simulink model "CubeX_LQR_2D"  (R2016b)
settings: Solver=FixedStepDiscrete  StartTime=0.0  StopTime=inf  FixedStep=Ts.base  RelTol=1e-3
PreLoadFcn:
  | waijung.modelPreload; % Required for working with Waijung Blockset. Do not remove.
InitFcn:
  | cubeparameters
  | LQR_2d
undefined symbols (not defined in the file): CPHA_1Edge, CPOL_Low, deg_, Duplex, FirstBit_MSB, Full, g, imu, K_lqr, Link, LQFP100, ST, STM32F407VG, STM32F4DISCOVERY, Ts
libraries: simulink x58, stm32f4_i2c_lib x12, stm32f4_io_lib x6, cube_lib x4, stm32f4_spi_lib x4, stm32f4_adc_lib x1, stm32f4_device_config_lib x1, BC_USB x1
(part 1 of 4)
CloseFcn:
  | waijung.modelClose; % Required for working with Waijung Blockset. Do not remove.
settings Model: Creator=Hi  LastModifiedBy=Wall
settings DataIOCC: LimitDataPoints=on  SaveFormat=Array
settings OptimizationCC: LifeSpan=1
settings DebuggingCC: AllowSymbolicDim=off  SFUnexpectedBacktrackingDiag=warning  SFNoUnconditionalDefaultTransitionDiag=warning  SFExecutionAtInitializationDiag=none
settings HardwareCC: ProdBitPerPointer=32  ProdBitPerSizeT=32  ProdBitPerPtrDiffT=32  ProdLargestAtomicFloat=None  ProdIntDivRoundTo=Undefined  ProdWordSize=32  ProdHWDeviceType=ARM Compatible->Cortex - M4  TargetEndianess=LittleEndian  TargetHWDeviceType=ARM Compatible->Cortex - M4
settings ModelReferenceCC: PropagateSignalLabelsOutOfModel=off
settings RTWCC: SystemTargetFile=stm32f4.tlc  GenerateMakefile=off  TemplateMakefile=ert_default_tmf  Description=STM32F4 Target
settings CodeAppCC: ForceParamTrailComments=on  IgnoreCustomStorageClasses=off  OperatorAnnotations=on  SimulinkDataObjDesc=on  InsertBlockDesc=on  MATLABSourceComments=on
settings STFCustomTargetCC: ModelReferenceCompliant=off  CombineOutputUpdateFcns=on  ERTCustomFileBanners=on  SupportContinuousTime=off  SupportNonInlinedSFcns=off  RemoveResetFunc=on  MATLABClassNameForMDSCustomization=Simulink.SoftwareTarget.ERTCustomization  GRTInterface=off  SystemTargetFile=stm32f4.tlc
settings ERTTargetCC: ModelReferenceCompliant=off  ParMdlRefBuildCompliant=off  CompOptLevelCompliant=off  ConcurrentExecutionCompliant=off  ERTFirstTimeCompliant=off  ModelStepFunctionPrototypeControlCompliant=off  CPPClassGenCompliant=off  UseToolchainInfoCompliant=off  ERTSrcFileBannerTemplate=stm32f4_code_template.cgt  ERTHdrFileBannerTemplate=stm32f4_code_template.cgt  ERTDataSrcFileTemplate=stm32f4_code_template.cgt  ERTDataHdrFileTemplate=stm32f4_code_template.cgt  ERTCustomFileTemplate=stm32f4_file_process.tlc  ConvertIfToSwitch=off  SuppressUnreachableDefaultCases=off
settings ConfigComp: CovMetricSettings=dw  CovHtmlReporting=on  CovSaveCumulativeToWorkspaceVar=on  CovSaveSingleToWorkspaceVar=on  CovExternalEMLEnable=off

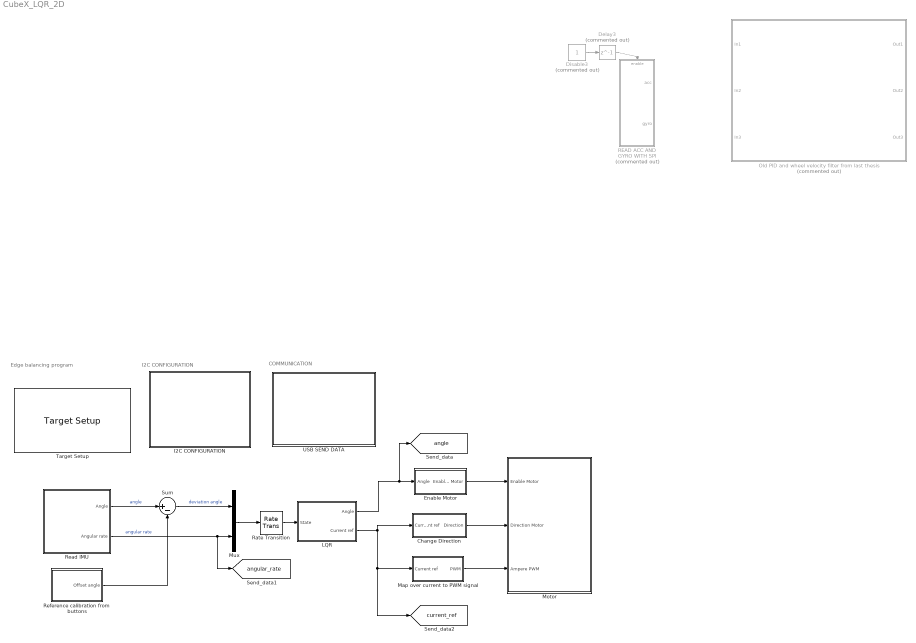
== system CubeX_LQR_2D ==
  note: Edge balancing program
  note: COMMUNICATION
  note: I2C CONFIGURATION
  Change Direction : Subsystem
  Delay3 : Delay  Commented=on  DelayLength=1  InitialCondition=0
  Disable3 : Constant  Commented=on
  Enable Motor : Subsystem  SystemSampleTime=Ts.controller
  I2C CONFIGURATION : Subsystem
  LQR : Subsystem  SystemSampleTime=Ts.controller
      settings: MinAlgLoopOccurrences=on
  Map over current to PWM signal : Subsystem
  Motor : Subsystem
  Mux : Mux  Inputs=2
  Old PID and wheel velocity filter from last thesis : Subsystem  Commented=on
  READ ACC AND GYRO WITH SPI : Subsystem  Commented=on
  Rate Transition : RateTransition  OutPortSampleTime=Ts.controller
  Read IMU : Subsystem
  Reference calibration from buttons : Subsystem
  Sum : Sum  Inputs=|+-
  Target Setup : stm32f4_device_config_lib/Target Setup  Priority=100  compiler=GNU ARM  previous_compiler=GNU ARM  mcu=STM32F407VG (LQFP100); STM32F4DISCOVERY  mcustr=STM32F407VG  clockconfig=STM32F4DISCOVERY Default (HSEOSC-8MHz/HCLK-168MHz)  system_stm32f4xx_c_path=C:\waijung15_04a\targets\stm32f4_target\stm32f4\utils\STM32F4xx_AN3988_V1.0.1\stm32f4_default\hseosc8mhz  showmemoryconfiguration=off  stacksize=0x400  heapsize=0x200  enableautocompiledownload=on  fullchiperase=off  programmerinterface=ST-Link  editctrlstr=on  compilercontrolstr=$(patsubst %, -I%, .) -mcpu=cortex-m4 -mthumb -mthumb-interwork -mfloat-abi=hard -mfpu=fpv4-sp-d16 -ffast-math -Wall -Wextra -Ofast  assemblercontrolstr=$(patsubst %, -I%, .) -mcpu=cortex-m4 -mthumb -mthumb-interwork -mfloat-abi=hard -mfpu=fpv4-sp-d16 -ffast-math -Wall -Wextra -Ofast -Wa,-amhls=$(<:.s=.lst) -D__STACK_SIZE=$(STACK_SIZE) -D__HEAP_SIZE=$(HEAP_SIZE)  linkercontrolstr=-T$(LD_SCRIPT) -g -Wl,-Map=$(MAP),--cref,--no-warn-mismatch -mcpu=cortex-m4 -mthumb -mthumb-interwork -mfloat-abi=hard -mfpu=fpv4-sp-d16  runafterdownload=on  execprofile=None  profileruart=1  profilerbaud=115200  profilertxpin=Not used  profilerinitstr=0.002,168000000,336000,115200,0  manualsetsampletime=on  sampletime=0.002  blockid=TargetSetup1  systickreloadvalue=336000  hseval=8000000  lastprofileruart=1  hclk=168000000  flashorigin=0x8000000  flashlength=1M  ramorigin=0x20000000  ramlength=112k  useextram=off
  USB SEND DATA : Subsystem
  tag scope: angle=global, angular_rate=global, current_ref=global
  wires:
  Disable3/1 -> Delay3/1
  Delay3/1 -> READ ACC AND GYRO WITH SPI/Enable
  Read IMU/2(Angular rate) -> [angular_rate], Mux/2  "angular rate"
  Reference calibration from buttons/1(Offset angle) -> Sum/2
  Sum/1 -> Mux/1  "deviation angle"
  Read IMU/1(Angle) -> Sum/1  "angle"
  LQR/2(Current ref) -> [current_ref], Map over current to PWM signal/1(Current ref), Change Direction/1(Current ref)
  Map over current to PWM signal/1(PWM) -> Motor/3(Ampere PWM)
  Change Direction/1(Direction) -> Motor/2("Direction Motor ")
  Enable Motor/1(Enable Motor) -> Motor/1(Enable Motor)
  Mux/1 -> Rate Transition/1
  Rate Transition/1 -> LQR/1(State)
  LQR/1(Angle) -> [angle], Enable Motor/1(Angle)

== system CubeX_LQR_2D/Change Direction ==
  Current ref : Inport
  Compare To Zero : simulink/Logic and Bit Operations/Compare To Zero  relop=<=  OutDataTypeStr=boolean
  Logical Operator : Logic  Operator=NOT  AllPortsSameDT=off  OutDataTypeStr=boolean
  Direction : Outport
  wires:
  Compare To Zero/1 -> Logical Operator/1
  Current ref/1 -> Compare To Zero/1
  Logical Operator/1 -> Direction/1

== system CubeX_LQR_2D/Enable Motor ==
  note: When the angle is abs of 6 degrees, Motor is enabled
  Angle : Inport
  Abs1 : Abs
  Compare To Constant : simulink/Logic and Bit Operations/Compare To Constant  relop=<=  const=deg2rad(3)  OutDataTypeStr=boolean
  Enable Motor : Outport
  wires:
  Abs1/1 -> Compare To Constant/1
  Angle/1 -> Abs1/1
  Compare To Constant/1 -> Enable Motor/1

== system CubeX_LQR_2D/I2C CONFIGURATION ==
  I2C Master Setup1 : S-Function  FunctionName=stm32f4_i2c  Parameters=configuration,module,transfer,clkspeed,timeout,sdapin,sclpin,writecount,readcount,inputtypearray,outputtypearray,confstr,sampletime,sampletimestr,blockid  SFunctionDeploymentMode=off  EnableBusSupport=off  mask(stm32f4_i2c){configuration=Setup, module=3, lastmodule=3, transfer=Blocking, dutycycle=TLow/THigh = 2, clkspeed=400, timeout=25, writecount=0, readcount=0, sdapin=C9, sclpin=A8, waitwritetime=0, inputtypearray=[0], outputtypearray=[0], confstr=["C","9","A","8","1","3","4","2","I2C_DutyCycle_2","0","off"], sampletime=-1, sampletimestr=0.002, blockid=I2CCONFIGURATIONI2CMasterSetup1}
      mask prompts: module "I2C Module"; lastmodule "Last module"; transfer "Transfer mode"; dutycycle "Duty cycle in fast mode"; clkspeed "Clock speed (kHz)"; timeout "Timeout (ms)"; writecount "Bytes write count"; readcount "Bytes read count"; sdapin "SDA pin"; sclpin "SCL pin"; waitwritetime "Wait write time (ms), default is 0"; inputtypearray "Input type array"; outputtypearray "Output type array"; confstr "Configuration string"; sampletime "Sample time (sec)"; sampletimestr "Compiled sample time (sec) in string"
      mask init:
      | stm32f4_i2c_callback('init');
      mask Help: web(fullfile(waijungdocroot,'stm32f4_i2c_setup.htm'), '-browser')
      mask TypeOptions configuration: Setup | Transaction
      mask Callback configuration: stm32f4_i2c_callback('configuration');
      mask TypeOptions module: 1 | 2 | 3
      mask Callback module: stm32f4_i2c_callback('module');
      mask TypeOptions transfer: Blocking | Non-blocking
      mask TypeOptions dutycycle: TLow/THigh = 16/9 | TLow/THigh = 2
      mask Callback dutycycle: stm32f4_i2c_callback('dutycycle');
      mask Callback writecount: stm32f4_i2c_callback('writecount');
      mask Callback readcount: stm32f4_i2c_callback('readcount');
      mask TypeOptions sdapin: - | C9
      mask Callback sdapin: stm32f4_i2c_callback('sdapin');
      mask TypeOptions sclpin: - | A8
      mask Callback sclpin: stm32f4_i2c_callback('sclpin');
      mask Callback confstr: stm32f4_i2c_callback('confstr');
      mask Callback sampletime: stm32f4_i2c_callback('sampletime');
      mask Callback sampletimestr: stm32f4_i2c_callback('sampletimestr');
      mask Callback blockid: stm32f4_i2c_callback('blockid');
      mask Display: text(0.5, 0.5, 'Module: I2C3\nClock: 400kHz\nSDA/SCL Pin: C9/A8','ver','middle','hor','center');
  I2C Master Setup2 : S-Function  FunctionName=stm32f4_i2c  Parameters=configuration,module,transfer,clkspeed,timeout,sdapin,sclpin,writecount,readcount,inputtypearray,outputtypearray,confstr,sampletime,sampletimestr,blockid  SFunctionDeploymentMode=off  EnableBusSupport=off  mask(stm32f4_i2c){configuration=Setup, module=1, lastmodule=1, transfer=Blocking, dutycycle=TLow/THigh = 2, clkspeed=400, timeout=25, writecount=0, readcount=0, sdapin=B9, sclpin=B6, waitwritetime=0, inputtypearray=[0], outputtypearray=[0], confstr=["B","9","B","6","1","1","6","0","I2C_DutyCycle_2","0","off"], sampletime=-1, sampletimestr=0.002, blockid=I2CCONFIGURATIONI2CMasterSetup2}
      mask prompts: module "I2C Module"; lastmodule "Last module"; transfer "Transfer mode"; dutycycle "Duty cycle in fast mode"; clkspeed "Clock speed (kHz)"; timeout "Timeout (ms)"; writecount "Bytes write count"; readcount "Bytes read count"; sdapin "SDA pin"; sclpin "SCL pin"; waitwritetime "Wait write time (ms), default is 0"; inputtypearray "Input type array"; outputtypearray "Output type array"; confstr "Configuration string"; sampletime "Sample time (sec)"; sampletimestr "Compiled sample time (sec) in string"
      mask init:
      | stm32f4_i2c_callback('init');
      mask Help: web(fullfile(waijungdocroot,'stm32f4_i2c_setup.htm'), '-browser')
      mask TypeOptions configuration: Setup | Transaction
      mask Callback configuration: stm32f4_i2c_callback('configuration');
      mask TypeOptions module: 1 | 2 | 3
      mask Callback module: stm32f4_i2c_callback('module');
      mask TypeOptions transfer: Blocking | Non-blocking
      mask TypeOptions dutycycle: TLow/THigh = 16/9 | TLow/THigh = 2
      mask Callback dutycycle: stm32f4_i2c_callback('dutycycle');
      mask Callback writecount: stm32f4_i2c_callback('writecount');
      mask Callback readcount: stm32f4_i2c_callback('readcount');
      mask TypeOptions sdapin: - | B7 | B9
      mask Callback sdapin: stm32f4_i2c_callback('sdapin');
      mask TypeOptions sclpin: - | B6 | B8
      mask Callback sclpin: stm32f4_i2c_callback('sclpin');
      mask Callback confstr: stm32f4_i2c_callback('confstr');
      mask Callback sampletime: stm32f4_i2c_callback('sampletime');
      mask Callback sampletimestr: stm32f4_i2c_callback('sampletimestr');
      mask Callback blockid: stm32f4_i2c_callback('blockid');
      mask Display: text(0.5, 0.5, 'Module: I2C1\nClock: 400kHz\nSDA/SCL Pin: B9/B6','ver','middle','hor','center');

== system CubeX_LQR_2D/LQR ==
  note: State feedback
      |
      | u = -Kx
  State : Inport
  Delay : Delay  DelayLength=1
  Demux : Demux  Outputs=2
  Estimate COG offset : MATLAB Function  TreatAsAtomicUnit=on
  Gain : Gain  Gain=-K_lqr  Multiplication=Matrix(K*u) (u vector)
  Mux : Mux  Inputs=2
  Sum : Sum  Inputs=++|
  Angle : Outport
  Current ref : Outport  Port=2
  tag scope: cog=global
  wires:
  Gain/1 -> Current ref/1, Estimate COG offset/1(iref)
  Demux/2 -> Mux/2, Estimate COG offset/3(wx)
  State/1 -> Demux/1
  Mux/1 -> Gain/1
  Sum/1 -> Angle/1, Mux/1
  Estimate COG offset/1(y) -> Delay/1
  Demux/1 -> Sum/2, Estimate COG offset/2(phi)
  Delay/1 -> Sum/1, [cog]

== system CubeX_LQR_2D/Map over current to PWM signal ==
  note: Debug for static friction
  note: Map over current to duty
      | current limit: 0-4A
      | duty limit: 10-90%
      |
      | (90-10) / (4-0) = 20 -> k
      | 10 -> m
  Current ref : Inport
  Abs : Abs
  Add : Sum
  Constant : Constant  Value=0  OutDataTypeStr=single  SampleTime=Ts.controller
  Saturation on duty : Saturate  UpperLimit=90  LowerLimit=10  OutDataTypeStr=single
  Sum : Sum  Inputs=|++
  k : Gain  Gain=20
  m : Constant  Value=10  OutDataTypeStr=single  SampleTime=Ts.controller
  PWM : Outport
  wires:
  Saturation on duty/1 -> PWM/1
  Current ref/1 -> Abs/1
  Abs/1 -> k/1
  k/1 -> Add/1
  m/1 -> Add/2
  Add/1 -> Sum/1
  Sum/1 -> Saturation on duty/1
  Constant/1 -> Sum/2

== system CubeX_LQR_2D/Motor ==
  Enable Motor : Inport
  "Direction Motor " : Inport  Port=2
  Ampere PWM : Inport  Port=3
  Direction Motor 3 (green) : stm32f4_io_lib/Digital Output  use_bitband=on  port=D  speed=100  porttype=Push Pull  porttypestr=PP  use_pin0=off  use_pin1=off  use_pin2=off  use_pin3=off  use_pin4=off  use_pin5=off  use_pin6=off  use_pin7=off  use_pin8=off  use_pin9=off  use_pin10=off  use_pin11=on  use_pin12=off  use_pin13=off  use_pin14=off  use_pin15=off  pinstr=GPIO_Pin_11  usedpinarray="[0  0  0  0  0  0  0  0  0  0  0  1  0  0  0  0]"  bitbandingstr="#define Motor1DirectionMotor3green_D11 Peripheral_BB(GPIOD->ODR, 11)  /* Output pin */"  sampletime=-1  sampletimestr=0.016  blockid=Motor1DirectionMotor3green  enablecustomportlabel=off  globalinit=off  cinputportlabel=In1, In2  coutputportlabel=0
  Enable Motor 3(yellow) : stm32f4_io_lib/Digital Output  use_bitband=on  port=D  speed=100  porttype=Push Pull  porttypestr=PP  use_pin0=off  use_pin1=off  use_pin2=off  use_pin3=off  use_pin4=off  use_pin5=off  use_pin6=off  use_pin7=off  use_pin8=off  use_pin9=on  use_pin10=off  use_pin11=off  use_pin12=off  use_pin13=off  use_pin14=off  use_pin15=off  pinstr=GPIO_Pin_9  usedpinarray="[0  0  0  0  0  0  0  0  0  1  0  0  0  0  0  0]"  bitbandingstr="#define Motor1EnableMotor3yellow_D9 Peripheral_BB(GPIOD->ODR, 9)  /* Output pin */"  sampletime=-1  sampletimestr=0.016  blockid=Motor1EnableMotor3yellow  enablecustomportlabel=off  globalinit=off  cinputportlabel=In1, In2  coutputportlabel=0
  PWM Ampere motor 3 : S-Function  FunctionName=stm32f4_basicpwm_fixed  Parameters=timer,pwmperiod,uc3m_pwmperiod,ch1pin,ch2pin,ch3pin,ch4pin,sampletime,sampletimestr,blockid,apb,portstr,pinstr,pinmat,timarr,timprescale,chmat,polaritystr  SFunctionDeploymentMode=off  EnableBusSupport=off  mask(stm32f4_basicpwm_fixed){timer=2, pwmperiod=0.02, uc3m_pwmperiod=0.0002, polarity=Active High, polaritystr=TIM_OCPolarity_High, ch1pin=Not available - Do not use, ch2pin=Not available - Do not use, ch3pin=Not available - Do not use, ch4pin=A3, sampletime=-1, sampletimestr=0.016, blockid=Motor1PWMAmperemotor3, portpinstr=,,,A3, enablecustomportlabel=off, cinputportlabel=In1, In2, In3, In4, coutputportlabel=0, callbackgensrccode=off, apb=1, portstr=["A"], pinstr=["GPIO_Pin_3"], pinmat=[1 3], timarr=59999, timprescale=55, chmat=[4]}
      mask prompts: pwmperiod "PWM Period (seconds)"; uc3m_pwmperiod "PWM Signal Period (seconds)"; ch1pin "Channel 1"; ch2pin "Channel 2"; ch3pin "Channel 3"; ch4pin "Channel 4"; sampletime "Sample time (sec)"; sampletimestr "Compiled sample time (sec) in string"; portpinstr "Port pin string"; enablecustomportlabel "Enable custom port labels"; cinputportlabel "Custom input port labels (Ex. In1, In2, In3)"; coutputportlabel "Custom output port labels (Ex. Out1, Out2, Out3)"; callbackgensrccode "Gen source code from callback"; portstr "Port string"; pinstr "Pin string"; pinmat "Pin matrix"; timarr "Timer ARR"; timprescale "Timer PRESCALE"; chmat "Channel order"
      mask help:
      | This block implements basic Edge-aligned Pulse Width Modulation (PWM) generation.
      | All timers are 16-bit. The PWM period is fixed (per timer).
      |
      | This block was fixed by Sr Antonio
      mask init:
      | stm32f4_basicpwm_callback_fixed('init');
      mask Help: web(fullfile(waijungdocroot,'stm32f4_basicpwm.htm'),'-browser')
      mask TypeOptions timer: 1 | 2 | 3 | 4 | 5 | 8 | 9 | 10 | 11 | 12 | 13 | 14
      mask Callback timer: stm32f4_basicpwm_callback_fixed('timer');
      mask Callback pwmperiod: stm32f4_basicpwm_callback_fixed('pwmperiod');
      mask Callback uc3m_pwmperiod: stm32f4_basicpwm_callback_fixed('uc3m_pwmperiod');
      mask TypeOptions polarity: Active High | Active Low
      mask Callback polarity: stm32f4_basicpwm_callback_fixed('polarity');
      mask TypeOptions ch1pin: Not available - Do not use | A0 | A5
      mask Callback ch1pin: stm32f4_basicpwm_callback_fixed('ch1pin');
      mask TypeOptions ch2pin: Not available - Do not use | A1 | B3
      mask Callback ch2pin: stm32f4_basicpwm_callback_fixed('ch2pin');
      mask TypeOptions ch3pin: Not available - Do not use | A2 | B10
      mask Callback ch3pin: stm32f4_basicpwm_callback_fixed('ch3pin');
      mask TypeOptions ch4pin: Not available - Do not use | A3 | B11
      mask Callback ch4pin: stm32f4_basicpwm_callback_fixed('ch4pin');
      mask Callback sampletime: stm32f4_basicpwm_callback_fixed('sampletime');
      mask Callback sampletimestr: stm32f4_basicpwm_callback_fixed('sampletimestr');
      mask Callback blockid: stm32f4_basicpwm_callback_fixed('blockid');
      mask Callback enablecustomportlabel: stm32f4_basicpwm_callback_fixed('enablecustomportlabel')
      mask Display: text(0.95, 0.5, 'UC3M FIXED\nTimer: 2\nPolarity: Active High\nPeriod (sec): 0.0002\nTs (sec): -1','ver','middle','hor','right');port_label('input', 1,'CH4 (A3)')
  "Velocty wheel 3, analog in (Grey), PC1" : stm32f4_adc_lib/Regular ADC  Commented=on  adcmodule=3  outputdatatype=Single  prescaler=2  prescalerstr=ADC_Prescaler_Div2  chsamplingtime=Auto  chsamplingtimestr=ADC_SampleTime_480Cycles  read_an0=off  read_an1=off  read_an2=off  read_an3=off  read_an4=off  read_an5=off  read_an6=off  read_an7=off  read_an8=off  read_an9=off  read_an10=on  read_an11=off  read_an12=off  read_an13=off  read_an14=off  read_an15=off  read_an16=off  read_an17=off  read_an18=off  pinstr=GPIO_Pin_10  usedpinarray="[0  0  0  0  0  0  0  0  0  0  1  0  0  0  0  0  0  0  0]"  usedportidarray=[2]  usedpinidarray=[0]  usedpinidcount=1  sampletime=0.002  blockid=Motor3Veloctywheel3analoginGreyPC1  enablecustomportlabel=off  cinputportlabel=0  coutputportlabel=Out1, Out2
  wires:
  Ampere PWM/1 -> PWM Ampere motor 3/1
  "Direction Motor "/1 -> Direction Motor 3 (green)/1
  Enable Motor/1 -> Enable Motor 3(yellow)/1

== system CubeX_LQR_2D/Old PID and wheel velocity filter from last thesis ==
  In1 : Inport
  In2 : Inport  Port=2
  In3 : Inport  Port=3
  Filetered Wheel 3 : Subsystem  Commented=on
  "PID Motor 3 DONE " : Subsystem  Commented=on
  Out1 : Outport
  Out2 : Outport  Port=2
  Out3 : Outport  Port=3
  wires:
  In1/1 -> "PID Motor 3 DONE "/1("Welocity Wheel ")
  "PID Motor 3 DONE "/2("Direction_Motor_3 ") -> Out3/1
  In2/1 -> Filetered Wheel 3/1(In1)
  Filetered Wheel 3/1(Out1) -> Out2/1
  "PID Motor 3 DONE "/1(Motor_3_Out) -> Out1/1
  In3/1 -> "PID Motor 3 DONE "/2(Angle)

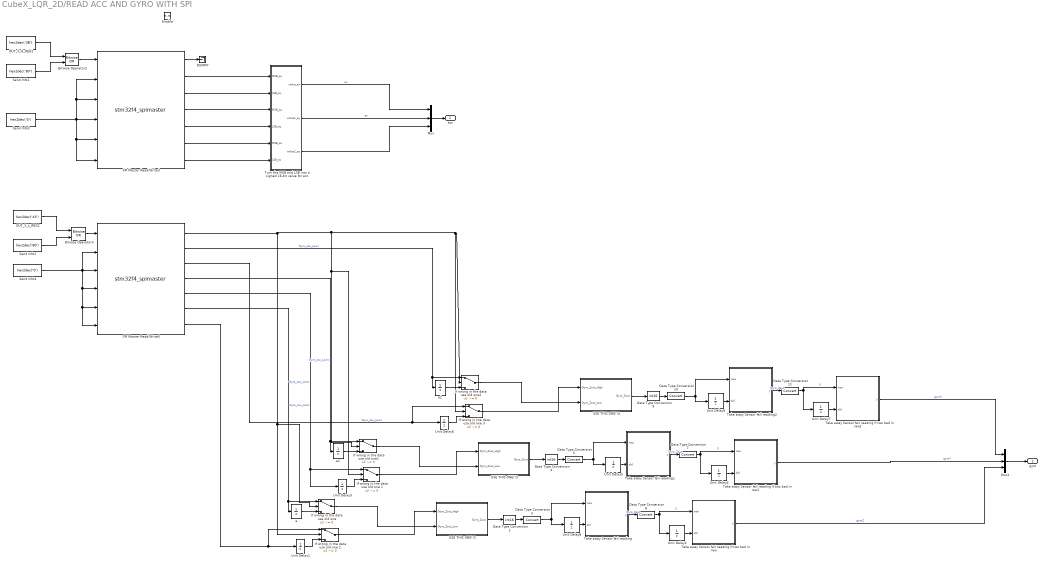
== system CubeX_LQR_2D/READ ACC AND GYRO WITH SPI ==
  Enable : EnablePort
  " a" : UnitDelay  SampleTime=-1
  " a1" : UnitDelay  SampleTime=-1
  " a2" : UnitDelay  SampleTime=-1
  Bitwise Operator2 : simulink/Logic and Bit Operations/Bitwise Operator  logicop=OR  UseBitMask=off  NumInputPorts=2  BitMask=bin2dec('11011001')  BitMaskRealWorld=Stored Integer
  Bitwise Operator3 : simulink/Logic and Bit Operations/Bitwise Operator  logicop=OR  UseBitMask=off  NumInputPorts=2  BitMask=bin2dec('11011001')  BitMaskRealWorld=Stored Integer
  DUMMY : Terminator
  Data Type Conversion{3,5,7..8,10..11} (6 alike) : DataTypeConversion
  Data Type Conversion2 : DataTypeConversion  OutDataTypeStr=int16
  Data Type Conversion4 : DataTypeConversion  OutDataTypeStr=int16
  Data Type Conversion9 : DataTypeConversion  OutDataTypeStr=int16
  If wrong in the data use old one : Switch  Criteria=u2 ~= 0
  If wrong in the data use old one 1 : Switch  Criteria=u2 ~= 0
  If wrong in the data use old one 2 : Switch  Criteria=u2 ~= 0
  If wrong in the data use old one 3 : Switch  Criteria=u2 ~= 0
  If wrong in the data use old one1 : Switch  Criteria=u2 ~= 0
  If wrong in the data use old one2 : Switch  Criteria=u2 ~= 0
  Mux : Mux  Inputs=3
  Mux1 : Mux  Inputs=3
  OUT_X_H_REG1 : Constant  Value=hex2dec('3B')  OutDataTypeStr=uint8
  OUT_X_L_REG2 : Constant  Value=hex2dec('43')  OutDataTypeStr=uint8
  SPI Master Read/Write3 : S-Function  FunctionName=stm32f4_spimaster  Parameters=mode,configuration,module,datacount,inputtypearray,outputtypearray,confstr,sampletime,sampletimestr,blockid  SFunctionDeploymentMode=off  EnableBusSupport=off  mask(stm32f4_spimaster){configuration=Transaction, module=3, mode=Read/ Write, lastmodule=1, direction=Full-Duplex, dataformat=8bit/ FirstBit_MSB, prescaler=4, cpolcpha=CPOL_Low/ CPHA_1Edge, datacount=6, nssmode=Custom, nsspin=Not used, softnssport=E, softnsspin=0, sckpin=A5, misopin=A6, mosipin=A7, inputtypearray=[6 3 3 3 3 3 3], outputtypearray=[7 7 3 3 3 3 3 3], confstr=["SPI_Direction_2Lines_FullDuplex","8b","MSB","Low","1Edge","4","Soft","0","x","x","0","x","x","1","A","5","1","A","6","1","A","7","1","0","0","0","0","0","0","0","0","PP","0","UP"], sampletime=-1, sampletimestr=Inf, blockid=SPI3getData4SPIMasterReadWrite3}
      mask prompts: module "SPI Module:"; lastmodule "Last module:"; dataformat "Data format:"; prescaler "Buad rate prescaler: Pclk/"; cpolcpha "Clock polarity (CPOL)/ Clock phase (CPHA):"; datacount "Data Read/Write count:"; nssmode "Slave/chip select (nSS, nCS) mode"; nsspin "Slave/chip select (nSS, nCS) pin"; softnssport "Slave/chip select port (nSS, nCS)"; softnsspin "Slave/chip select pin (nSS, nCS)"; sckpin "SCLK pin:"; misopin "MISO pin:"; mosipin "MOSI pin:"; inputtypearray "Input type array"; outputtypearray "Output type array"; confstr "Configuration string"; sampletime "Sample time (sec)"; sampletimestr "Compiled sample time (sec) in string"
      mask help:
      | Status:
      |  0 - Success.
      |  Otherwise - Fail.
      mask init:
      | stm32f4_spimaster_callback('init');
      mask Help: web(fullfile(waijungdocroot,'stm32f4_spimaster_readwrite.htm'), '-browser')
      mask TypeOptions configuration: Setup | Transaction
      mask Callback configuration: stm32f4_spimaster_callback('configuration');
      mask TypeOptions module: 1 | 2 | 3
      mask Callback module: stm32f4_spimaster_callback('module');
      mask TypeOptions mode: Read/ Write | Read | Write
      mask Callback mode: stm32f4_spimaster_callback('mode');
      mask TypeOptions direction: Full-Duplex | Half-Duplex_Tx | Half-Duplex_Rx
      mask Callback direction: stm32f4_spimaster_callback('direction');
      mask TypeOptions dataformat: 8bit/ FirstBit_MSB | 8bit/ FirstBit_LSB | 16bit/ FirstBit_MSB | 16bit/ FirstBit_LSB
      mask TypeOptions prescaler: 2 | 4 | 8 | 16 | 32 | 64 | 128 | 256
      mask TypeOptions cpolcpha: CPOL_Low/ CPHA_1Edge | CPOL_Low/ CPHA_2Edge | CPOL_High/ CPHA_1Edge | CPOL_High/ CPHA_2Edge
      mask Callback datacount: stm32f4_spimaster_callback('datacount');
      mask TypeOptions nssmode: Hardware | Software | Custom
      mask Callback nssmode: stm32f4_spimaster_callback('nssmode');
      mask TypeOptions nsspin: Not used | A4 | A15
      mask TypeOptions softnssport: A | B | C | D | E | F | G | H | I
      mask TypeOptions softnsspin: 0 | 1 | 2 | 3 | 4 | 5 | 6 | 7 | 8 | 9 | 10 | 11 | 12 | 13 | 14 | 15
      mask TypeOptions sckpin: Not used | A5 | B3
      mask TypeOptions misopin: Not used | A6 | B4
      mask TypeOptions mosipin: Not used | A7 | B5
      mask Callback confstr: stm32f4_spimaster_callback('confstr');
      mask Callback sampletime: stm32f4_spimaster_callback('sampletime');
      mask Callback sampletimestr: stm32f4_spimaster_callback('sampletimestr');
      mask Callback blockid: stm32f4_spimaster_callback('blockid');
      mask Display: text(0.5, 0.5, 'Module: SPI3 (Master)\nRead/ Write\nTs (sec): Inf','ver','middle','hor','center');port_label('input', 1,'Wr0 (uint8)');port_label('input', 2,'Wr1 (uint8)');port_label('input', 3,'Wr2 (uint8)');port_label('input', 4,'Wr3 (uint8)');port_label('input', 5,'Wr4 (uint8)');port_label('input', 6,'Wr5 (uint8)');port_label('output', 1,'Status');port_label('output', 2,'Rd0 (uint8)');port_label('output', 3,'Rd1 (uint8)');port_label('output', 4,'Rd2 (uint8)');port_label('output', 5,'Rd3 (uint8)');port_label('output', 6,'Rd4 (uint8)');port_label('output', 7,'Rd5 (uint8)');
  SPI Master Read/Write5 : S-Function  FunctionName=stm32f4_spimaster  Parameters=mode,configuration,module,datacount,inputtypearray,outputtypearray,confstr,sampletime,sampletimestr,blockid  SFunctionDeploymentMode=off  EnableBusSupport=off  mask(stm32f4_spimaster){configuration=Transaction, module=3, mode=Read/ Write, lastmodule=1, direction=Full-Duplex, dataformat=8bit/ FirstBit_MSB, prescaler=4, cpolcpha=CPOL_Low/ CPHA_1Edge, datacount=6, nssmode=Custom, nsspin=Not used, softnssport=E, softnsspin=0, sckpin=A5, misopin=A6, mosipin=A7, inputtypearray=[6 3 3 3 3 3 3], outputtypearray=[7 7 3 3 3 3 3 3], confstr=["SPI_Direction_2Lines_FullDuplex","8b","MSB","Low","1Edge","4","Soft","0","x","x","0","x","x","1","A","5","1","A","6","1","A","7","1","0","0","0","0","0","0","0","0","PP","0","UP"], sampletime=-1, sampletimestr=Inf, blockid=SPI3getData4SPIMasterReadWrite5}
      mask prompts: module "SPI Module:"; lastmodule "Last module:"; dataformat "Data format:"; prescaler "Buad rate prescaler: Pclk/"; cpolcpha "Clock polarity (CPOL)/ Clock phase (CPHA):"; datacount "Data Read/Write count:"; nssmode "Slave/chip select (nSS, nCS) mode"; nsspin "Slave/chip select (nSS, nCS) pin"; softnssport "Slave/chip select port (nSS, nCS)"; softnsspin "Slave/chip select pin (nSS, nCS)"; sckpin "SCLK pin:"; misopin "MISO pin:"; mosipin "MOSI pin:"; inputtypearray "Input type array"; outputtypearray "Output type array"; confstr "Configuration string"; sampletime "Sample time (sec)"; sampletimestr "Compiled sample time (sec) in string"
      mask help:
      | Status:
      |  0 - Success.
      |  Otherwise - Fail.
      mask init:
      | stm32f4_spimaster_callback('init');
      mask Help: web(fullfile(waijungdocroot,'stm32f4_spimaster_readwrite.htm'), '-browser')
      mask TypeOptions configuration: Setup | Transaction
      mask Callback configuration: stm32f4_spimaster_callback('configuration');
      mask TypeOptions module: 1 | 2 | 3
      mask Callback module: stm32f4_spimaster_callback('module');
      mask TypeOptions mode: Read/ Write | Read | Write
      mask Callback mode: stm32f4_spimaster_callback('mode');
      mask TypeOptions direction: Full-Duplex | Half-Duplex_Tx | Half-Duplex_Rx
      mask Callback direction: stm32f4_spimaster_callback('direction');
      mask TypeOptions dataformat: 8bit/ FirstBit_MSB | 8bit/ FirstBit_LSB | 16bit/ FirstBit_MSB | 16bit/ FirstBit_LSB
      mask TypeOptions prescaler: 2 | 4 | 8 | 16 | 32 | 64 | 128 | 256
      mask TypeOptions cpolcpha: CPOL_Low/ CPHA_1Edge | CPOL_Low/ CPHA_2Edge | CPOL_High/ CPHA_1Edge | CPOL_High/ CPHA_2Edge
      mask Callback datacount: stm32f4_spimaster_callback('datacount');
      mask TypeOptions nssmode: Hardware | Software | Custom
      mask Callback nssmode: stm32f4_spimaster_callback('nssmode');
      mask TypeOptions nsspin: Not used | A4 | A15
      mask TypeOptions softnssport: A | B | C | D | E | F | G | H | I
      mask TypeOptions softnsspin: 0 | 1 | 2 | 3 | 4 | 5 | 6 | 7 | 8 | 9 | 10 | 11 | 12 | 13 | 14 | 15
      mask TypeOptions sckpin: Not used | A5 | B3
      mask TypeOptions misopin: Not used | A6 | B4
      mask TypeOptions mosipin: Not used | A7 | B5
      mask Callback confstr: stm32f4_spimaster_callback('confstr');
      mask Callback sampletime: stm32f4_spimaster_callback('sampletime');
      mask Callback sampletimestr: stm32f4_spimaster_callback('sampletimestr');
      mask Callback blockid: stm32f4_spimaster_callback('blockid');
      mask Display: text(0.5, 0.5, 'Module: SPI3 (Master)\nRead/ Write\nTs (sec): Inf','ver','middle','hor','center');port_label('input', 1,'Wr0 (uint8)');port_label('input', 2,'Wr1 (uint8)');port_label('input', 3,'Wr2 (uint8)');port_label('input', 4,'Wr3 (uint8)');port_label('input', 5,'Wr4 (uint8)');port_label('input', 6,'Wr5 (uint8)');port_label('output', 1,'Status');port_label('output', 2,'Rd0 (uint8)');port_label('output', 3,'Rd1 (uint8)');port_label('output', 4,'Rd2 (uint8)');port_label('output', 5,'Rd3 (uint8)');port_label('output', 6,'Rd4 (uint8)');port_label('output', 7,'Rd5 (uint8)');
  Send Info1 : Constant  Value=hex2dec('80')  OutDataTypeStr=uint8
  Send Info2 : Constant  Value=hex2dec('80')  OutDataTypeStr=uint8
  Send Info3 : Constant  Value=hex2dec('0')  OutDataTypeStr=uint8
  Send Info4 : Constant  Value=hex2dec('0')  OutDataTypeStr=uint8
  Take away Sensor fail reading : MATLAB Function  TreatAsAtomicUnit=on
  Take away Sensor fail reading if two bad in raw : MATLAB Function  TreatAsAtomicUnit=on
  Take away Sensor fail reading if two bad in raw1 : MATLAB Function  TreatAsAtomicUnit=on
  Take away Sensor fail reading if two bad in raw2 : MATLAB Function  TreatAsAtomicUnit=on
  Take away Sensor fail reading1 : MATLAB Function  TreatAsAtomicUnit=on
  Take away Sensor fail reading2 : MATLAB Function  TreatAsAtomicUnit=on
  Turn the MSB and LSB into a signed 16-bit value for acc : Subsystem
  USE THIS ONE!!2 : Subsystem
  USE THIS ONE!!3 : Subsystem
  USE THIS ONE!!4 : Subsystem
  Unit Delay1 : UnitDelay  SampleTime=-1
  Unit Delay{2,4..5,7..9} (6 alike) : UnitDelay  InitialCondition=-40.45  SampleTime=-1
  Unit Delay3 : UnitDelay  SampleTime=-1
  Unit Delay6 : UnitDelay  SampleTime=-1
  acc : Outport
  gyro : Outport  Port=2
  wires:
  Bitwise Operator3/1 -> SPI Master Read/Write5/1
  OUT_X_H_REG1/1 -> Bitwise Operator2/1
  OUT_X_L_REG2/1 -> Bitwise Operator3/1
  Send Info2/1 -> Bitwise Operator3/2
  Bitwise Operator2/1 -> SPI Master Read/Write3/1
  Send Info1/1 -> Bitwise Operator2/2
  Send Info4/1 -> SPI Master Read/Write5/2, SPI Master Read/Write5/6, SPI Master Read/Write5/5, SPI Master Read/Write5/4, SPI Master Read/Write5/3
  SPI Master Read/Write3/1 -> DUMMY/1
  USE THIS ONE!!2/1(Gyro_Zout) -> Data Type Conversion2/1
  Data Type Conversion2/1 -> Data Type Conversion3/1
  SPI Master Read/Write5/6 -> " a"/1, If wrong in the data use old one/1  "Gyro_zou_Lowt"
  " a"/1 -> If wrong in the data use old one/3
  SPI Master Read/Write5/7 -> If wrong in the data use old one 2/1, Unit Delay1/1
  Unit Delay1/1 -> If wrong in the data use old one 2/3
  If wrong in the data use old one/1 -> USE THIS ONE!!2/2(Gyro_Zout_Low)
  If wrong in the data use old one 2/1 -> USE THIS ONE!!2/1("Gyro_Zout_High ")
  Unit Delay8/1 -> Take away Sensor fail reading/2(old)
  Take away Sensor fail reading/1(y) -> Data Type Conversion8/1  "Gyro_Zout"
  Unit Delay2/1 -> Take away Sensor fail reading if two bad in raw/2(old)
  Data Type Conversion8/1 -> Unit Delay2/1, Take away Sensor fail reading if two bad in raw/1(new)  "3"
  Take away Sensor fail reading if two bad in raw/1(y) -> Mux1/3  "gyroZ"
  Data Type Conversion3/1 -> Take away Sensor fail reading/1(new), Unit Delay8/1
  SPI Master Read/Write5/3 -> If wrong in the data use old one 3/1, Unit Delay6/1  "Gyro_zou_Lowt"
  SPI Master Read/Write5/5 -> Unit Delay3/1, If wrong in the data use old one 1/1  "Gyro_zou_Lowt"
  USE THIS ONE!!3/1(Gyro_Zout) -> Data Type Conversion4/1
  Data Type Conversion4/1 -> Data Type Conversion5/1
  SPI Master Read/Write5/4 -> " a1"/1, If wrong in the data use old one1/1  "Gyro_zou_Lowt"
  " a1"/1 -> If wrong in the data use old one1/3
  Unit Delay3/1 -> If wrong in the data use old one 1/3
  If wrong in the data use old one1/1 -> USE THIS ONE!!3/2(Gyro_Zout_Low)
  If wrong in the data use old one 1/1 -> USE THIS ONE!!3/1("Gyro_Zout_High ")
  Unit Delay5/1 -> Take away Sensor fail reading1/2(old)
  Take away Sensor fail reading1/1(y) -> Data Type Conversion7/1  "Gyro_Zout"
  Unit Delay4/1 -> Take away Sensor fail reading if two bad in raw1/2(old)
  Data Type Conversion7/1 -> Unit Delay4/1, Take away Sensor fail reading if two bad in raw1/1(new)  "3"
  Data Type Conversion5/1 -> Take away Sensor fail reading1/1(new), Unit Delay5/1
  USE THIS ONE!!4/1(Gyro_Zout) -> Data Type Conversion9/1
  Data Type Conversion9/1 -> Data Type Conversion10/1
  SPI Master Read/Write5/2 -> " a2"/1, If wrong in the data use old one2/1  "Gyro_zou_Lowt"
  " a2"/1 -> If wrong in the data use old one2/3
  Unit Delay6/1 -> If wrong in the data use old one 3/3
  If wrong in the data use old one2/1 -> USE THIS ONE!!4/2(Gyro_Zout_Low)
  If wrong in the data use old one 3/1 -> USE THIS ONE!!4/1("Gyro_Zout_High ")
  Unit Delay9/1 -> Take away Sensor fail reading2/2(old)
  Take away Sensor fail reading2/1(y) -> Data Type Conversion11/1  "Gyro_Zout"
  Unit Delay7/1 -> Take away Sensor fail reading if two bad in raw2/2(old)
  Data Type Conversion11/1 -> Unit Delay7/1, Take away Sensor fail reading if two bad in raw2/1(new)  "3"
  Take away Sensor fail reading if two bad in raw2/1(y) -> Mux1/1  "gyroX"
  Data Type Conversion10/1 -> Take away Sensor fail reading2/1(new), Unit Delay9/1
  SPI Master Read/Write5/1 -> If wrong in the data use old one2/2, If wrong in the data use old one 3/2, If wrong in the data use old one 1/2, If wrong in the data use old one1/2, If wrong in the data use old one 2/2, If wrong in the data use old one/2
  Send Info3/1 -> SPI Master Read/Write3/2, SPI Master Read/Write3/3, SPI Master Read/Write3/4, SPI Master Read/Write3/5, SPI Master Read/Write3/6
  Mux/1 -> acc/1
  Turn the MSB and LSB into a signed 16-bit value for acc/1(value_ax) -> Mux/1  "ax"
  Turn the MSB and LSB into a signed 16-bit value for acc/2(value1_ay) -> Mux/2  "ay"
  Mux1/1 -> gyro/1
  Take away Sensor fail reading if two bad in raw1/1(y) -> Mux1/2  "gyroY"
  SPI Master Read/Write3/6 -> Turn the MSB and LSB into a signed 16-bit value for acc/5(MSB_az)
  SPI Master Read/Write3/7 -> Turn the MSB and LSB into a signed 16-bit value for acc/6(LSB_az)
  SPI Master Read/Write3/2 -> Turn the MSB and LSB into a signed 16-bit value for acc/1(MSB_ax)
  SPI Master Read/Write3/3 -> Turn the MSB and LSB into a signed 16-bit value for acc/2("LSB_ax ")
  SPI Master Read/Write3/4 -> Turn the MSB and LSB into a signed 16-bit value for acc/3(MSB_ay)
  SPI Master Read/Write3/5 -> Turn the MSB and LSB into a signed 16-bit value for acc/4(LSB_ay)
  Turn the MSB and LSB into a signed 16-bit value for acc/3(value2_az) -> Mux/3

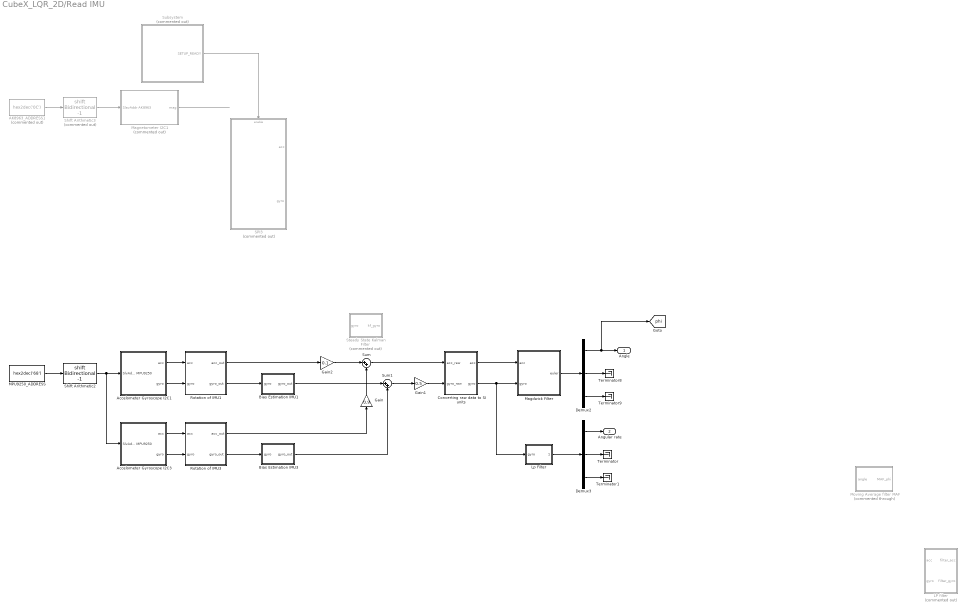
== system CubeX_LQR_2D/Read IMU ==
  " AK8963_ADDRESS1" : Constant  Commented=on  Value=hex2dec('0C')  OutDataTypeStr=uint8  SampleTime=0.002
  " MPU9250_ADDRESS" : Constant  Value=hex2dec('68')  OutDataTypeStr=uint8  SampleTime=Ts.IMU
  Accelometer Gyroscope I2C1 : Subsystem
  Accelometer Gyroscope I2C3 : Subsystem
  Bias Estimation IMU1 : MATLAB Function  TreatAsAtomicUnit=on
  Bias Estimation IMU3 : MATLAB Function  TreatAsAtomicUnit=on
  Converting raw data to SI units : Subsystem
  Demux2 : Demux  Outputs=3
  Demux3 : Demux  Outputs=3
  Gain : Gain  Gain=0.9
  Gain1 : Gain  Gain=0.5
  Gain2 : Gain  Gain=0.1
  LP filter : MATLAB Function  Commented=on  TreatAsAtomicUnit=on
  Lp Filter : MATLAB Function  TreatAsAtomicUnit=on
  Magdwick Filter : MATLAB Function  TreatAsAtomicUnit=on
  Magnetometer I2C1 : Subsystem  Commented=on
  Moving Average filter MAF : MATLAB Function  Commented=through  TreatAsAtomicUnit=on
  Rotation of IMU1 : MATLAB Function  TreatAsAtomicUnit=on
  Rotation of IMU3 : MATLAB Function  TreatAsAtomicUnit=on
  SPI3 : Subsystem  Commented=on
  Shift Arithmetic2 : ArithShift  BitShiftNumber=-1
  Shift Arithmetic3 : ArithShift  Commented=on  BitShiftNumber=-1
  Steady State Kalman Filter : MATLAB Function  Commented=on  TreatAsAtomicUnit=on
  Subsystem : Subsystem  Commented=on
  Sum : Sum  Inputs=|++
  Sum1 : Sum  Inputs=|++
  Terminator{,1,8..9} (4 alike) : Terminator
  Angle : Outport
  Angular rate : Outport  Port=2
  tag scope: phi=global
  wires:
  Demux3/2 -> Terminator/1
  Demux2/2 -> Terminator8/1
  Demux2/3 -> Terminator9/1
  Demux3/3 -> Terminator1/1
  Converting raw data to SI units/1(acc) -> Magdwick Filter/1(acc)
  Demux3/1 -> Angular rate/1
  Magdwick Filter/1(euler) -> Demux2/1
  Accelometer Gyroscope I2C1/2(gyro) -> Rotation of IMU1/2(gyro)
  Subsystem/1(SETUP_READY) -> SPI3/Enable
  Shift Arithmetic2/1 -> Accelometer Gyroscope I2C3/1(SlvAddr MPU9250), Accelometer Gyroscope I2C1/1(SlvAddr MPU9250)
  Accelometer Gyroscope I2C1/1(acc) -> Rotation of IMU1/1(acc)
  " MPU9250_ADDRESS"/1 -> Shift Arithmetic2/1
  Shift Arithmetic3/1 -> Magnetometer I2C1/1(SlavAddr AK8963)
  " AK8963_ADDRESS1"/1 -> Shift Arithmetic3/1
  Magnetometer I2C1/1(mag) -> ?
  Accelometer Gyroscope I2C3/1(acc) -> Rotation of IMU3/1(acc)
  Accelometer Gyroscope I2C3/2(gyro) -> Rotation of IMU3/2(gyro)
  Rotation of IMU1/2(gyro_out) -> Bias Estimation IMU1/1(gyro)
  Rotation of IMU3/2(gyro_out) -> Bias Estimation IMU3/1(gyro)
  Sum1/1 -> Gain1/1
  Sum/1 -> Converting raw data to SI units/1(acc_raw)
  Bias Estimation IMU1/1(gyro_out) -> Sum1/1
  Gain2/1 -> Sum/1
  Gain/1 -> Sum/2
  Gain1/1 -> Converting raw data to SI units/2(gyro_raw)
  Bias Estimation IMU3/1(gyro_out) -> Sum1/2
  Rotation of IMU3/1(acc_out) -> Gain/1
  Rotation of IMU1/1(acc_out) -> Gain2/1
  Demux2/1 -> [phi], Angle/1
  Lp Filter/1(filter_gyro) -> Demux3/1
  Converting raw data to SI units/2(gyro) -> Lp Filter/1(gyro), Magdwick Filter/2(gyro)

== system CubeX_LQR_2D/Reference calibration from buttons ==
  Calibration Minus : stm32f4_io_lib/Digital Input  port=E  speed=100  porttype=Pull Up  porttypestr=UP  use_pin0=off  use_pin1=off  use_pin2=off  use_pin3=off  use_pin4=off  use_pin5=off  use_pin6=off  use_pin7=off  use_pin8=off  use_pin9=off  use_pin10=off  use_pin11=off  use_pin12=off  use_pin13=off  use_pin14=on  use_pin15=off  pinstr=GPIO_Pin_14  usedpinarray="[0  0  0  0  0  0  0  0  0  0  0  0  0  0  1  0]"  bitbandingstr="#define ReferencecalibrationfrombuttonsCalibrationMinus_E14 Peripheral_BB(GPIOE->IDR, 14)  /* Output pin */"  sampletime=Ts.IMU  sampletimestr=0.008  blockid=ReferencecalibrationfrombuttonsCalibrationMinus  enablecustomportlabel=off  glabalinit=off  cinputportlabel=In1, In2  coutputportlabel=Out1, Out2
  Calibration Plus : stm32f4_io_lib/Digital Input  port=E  speed=100  porttype=Pull Up  porttypestr=UP  use_pin0=off  use_pin1=off  use_pin2=off  use_pin3=off  use_pin4=off  use_pin5=off  use_pin6=off  use_pin7=off  use_pin8=off  use_pin9=off  use_pin10=off  use_pin11=on  use_pin12=off  use_pin13=off  use_pin14=off  use_pin15=off  pinstr=GPIO_Pin_11  usedpinarray="[0  0  0  0  0  0  0  0  0  0  0  1  0  0  0  0]"  bitbandingstr="#define ReferencecalibrationfrombuttonsCalibrationPlus_E11 Peripheral_BB(GPIOE->IDR, 11)  /* Output pin */"  sampletime=Ts.IMU  sampletimestr=0.008  blockid=ReferencecalibrationfrombuttonsCalibrationPlus  enablecustomportlabel=off  glabalinit=off  cinputportlabel=In1, In2  coutputportlabel=Out1, Out2
  Compare To Constant10 : simulink/Logic and Bit Operations/Compare To Constant  relop===  const=0  OutDataTypeStr=boolean  ZeroCross=off
  Compare To Constant2 : simulink/Logic and Bit Operations/Compare To Constant  relop===  const=0  OutDataTypeStr=boolean  ZeroCross=off
  Constant : Constant  Value=48.08  OutDataTypeStr=single  SampleTime=Ts.IMU
  Reference calibration calculation : MATLAB Function  TreatAsAtomicUnit=on
  Rising edge boolean1 : cube_lib/Rising edge boolean
  Rising edge boolean2 : cube_lib/Rising edge boolean
  deg2rad : Gain  Gain=pi/180  ParamDataTypeStr=single
  Offset angle : Outport
  wires:
  Compare To Constant10/1 -> Rising edge boolean2/1
  Reference calibration calculation/1(correction_out) -> deg2rad/1
  Calibration Minus/1 -> Compare To Constant2/1
  Calibration Plus/1 -> Compare To Constant10/1
  Rising edge boolean1/1 -> Reference calibration calculation/2(ref_minus)
  Compare To Constant2/1 -> Rising edge boolean1/1
  Rising edge boolean2/1 -> Reference calibration calculation/1(ref_plus)
  Constant/1 -> Reference calibration calculation/3(inital_offset)
  deg2rad/1 -> Offset angle/1

== system CubeX_LQR_2D/USB SEND DATA ==
  USB VCP Send STM32F1 : BC_USB/USB VCP Send STM32F4  speed="USB 1.1   12Mbit/s"  data_size=2048 Bytes  header_data='0E 0E'  binary_data='single single single single'  terminator_data='0A 0A'  sampletime=Ts.base
  wires:
  [angle] -> USB VCP Send STM32F1/1
  [angular_rate] -> USB VCP Send STM32F1/2
  [current_ref] -> USB VCP Send STM32F1/3
  [cog] -> USB VCP Send STM32F1/4

== system CubeX_LQR_2D/Old PID and wheel velocity filter from last thesis/Filetered Wheel 3 ==
  In1 : Inport
  Add3 : Sum  Inputs=-+
  Add9 : Sum  Inputs=-+
  Constant1 : Constant  Value=2094  SampleTime=-1
  Constant15 : Constant  Value=69  SampleTime=-1
  Gain2 : Gain  Gain=(6110*2)/4096
  RPM to RAD3 : Gain  Gain=1/9.55
  Scope : Scope
  Out1 : Outport
  wires:
  Gain2/1 -> RPM to RAD3/1
  Add3/1 -> Gain2/1
  Constant1/1 -> Add3/1
  In1/1 -> Add3/2
  Constant15/1 -> Add9/1
  RPM to RAD3/1 -> Add9/2
  Add9/1 -> Scope/1, Out1/1

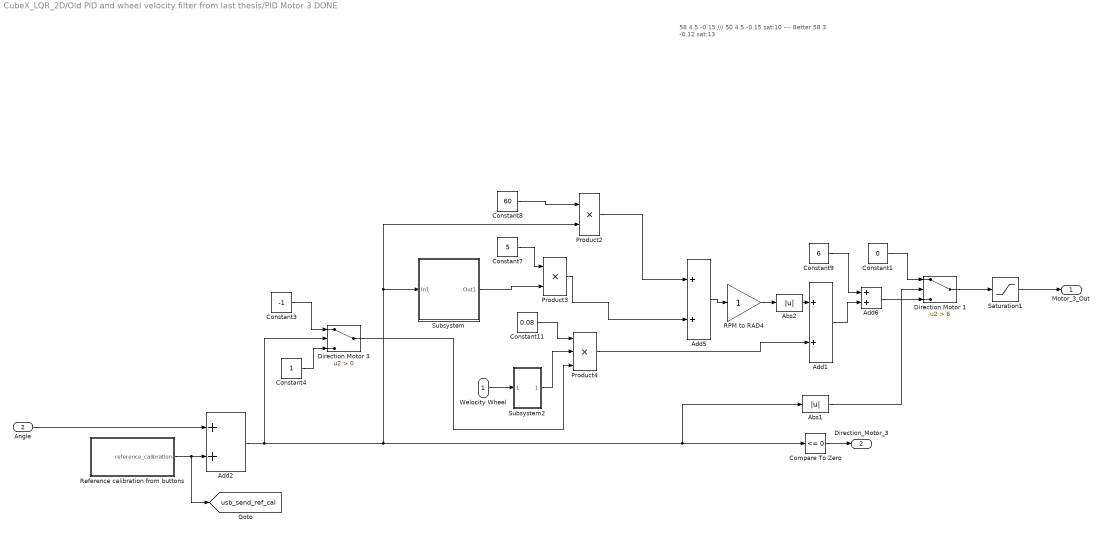
== system CubeX_LQR_2D/Old PID and wheel velocity filter from last thesis/PID Motor 3 DONE  ==
  note: 58
      | 4.5
      | -0.15
      | ///
      | 50
      | 4.5
      | -0.15
      | sat:10
      | --- Better
      | 58
      | 3
      | -0.12
      | sat:13
  "Welocity Wheel " : Inport
  Angle : Inport  Port=2
  Abs1 : Abs
  Abs2 : Abs
  Add{1..2,5..6} (4 alike) : Sum
  Compare To Zero : simulink/Logic and Bit Operations/Compare To Zero  relop=<=  OutDataTypeStr=boolean
  Constant1 : Constant  Value=0  OutDataTypeStr=single  SampleTime=-1
  Constant11 : Constant  Value=0.08  OutDataTypeStr=single  SampleTime=-1
  Constant3 : Constant  Value=-1  OutDataTypeStr=single  SampleTime=-1
  Constant4 : Constant  OutDataTypeStr=single  SampleTime=-1
  Constant7 : Constant  Value=5  OutDataTypeStr=single  SampleTime=-1
  Constant8 : Constant  Value=60  OutDataTypeStr=single  SampleTime=-1
  Constant9 : Constant  Value=6  SampleTime=-1
  Direction Motor 1 : Switch  Criteria=u2 > Threshold  Threshold=6
  Direction Motor 3 : Switch  Criteria=u2 > Threshold
  Product2 : Product
  Product3 : Product
  Product4 : Product  Inputs=3
  RPM to RAD4 : Gain
  Reference calibration from buttons : Subsystem
  Saturation1 : Saturate  UpperLimit=90  LowerLimit=10
  Subsystem : Subsystem
  Subsystem2 : Subsystem
  Motor_3_Out : Outport
  "Direction_Motor_3 " : Outport  Port=2
  tag scope: usb_send_ref_cal=global
  wires:
  Compare To Zero/1 -> "Direction_Motor_3 "/1
  Constant7/1 -> Product3/1
  Constant11/1 -> Product4/1
  Product3/1 -> Add5/2
  Constant9/1 -> Add6/1
  Add5/1 -> RPM to RAD4/1
  RPM to RAD4/1 -> Abs2/1
  Product2/1 -> Add5/1
  Abs2/1 -> Add1/1
  Saturation1/1 -> Motor_3_Out/1
  Constant8/1 -> Product2/1
  Add6/1 -> Direction Motor 1/3
  Direction Motor 1/1 -> Saturation1/1
  Constant1/1 -> Direction Motor 1/1
  Abs1/1 -> Direction Motor 1/2
  Product4/1 -> Add1/2
  "Welocity Wheel "/1 -> Subsystem2/1(In1)
  Angle/1 -> Add2/1
  Subsystem/1(Out1) -> Product3/2
  Add1/1 -> Add6/2
  Constant4/1 -> Direction Motor 3/3
  Constant3/1 -> Direction Motor 3/1
  Direction Motor 3/1 -> Product4/3
  Subsystem2/1(Out2) -> Product4/2
  Reference calibration from buttons/1(reference_calibration) -> [usb_send_ref_cal], Add2/2
  Add2/1 -> Direction Motor 3/2, Subsystem/1(In1), Product2/2, Compare To Zero/1, Abs1/1

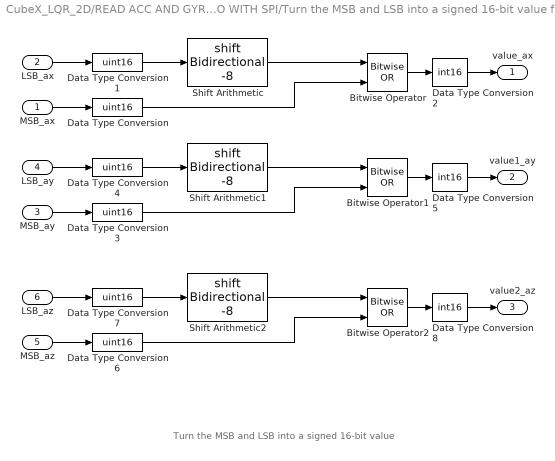
== system CubeX_LQR_2D/READ ACC AND GYRO WITH SPI/Turn the MSB and LSB into a signed 16-bit value for acc ==
  note: Turn the MSB and LSB into a signed 16-bit value
  MSB_ax : Inport
  "LSB_ax " : Inport  Port=2
  MSB_ay : Inport  Port=3
  LSB_ay : Inport  Port=4
  MSB_az : Inport  Port=5
  LSB_az : Inport  Port=6
  Bitwise Operator : simulink/Logic and Bit Operations/Bitwise Operator  logicop=OR  UseBitMask=off  NumInputPorts=2  BitMask=bin2dec('11011001')  BitMaskRealWorld=Stored Integer
  Bitwise Operator1 : simulink/Logic and Bit Operations/Bitwise Operator  logicop=OR  UseBitMask=off  NumInputPorts=2  BitMask=bin2dec('11011001')  BitMaskRealWorld=Stored Integer
  Bitwise Operator2 : simulink/Logic and Bit Operations/Bitwise Operator  logicop=OR  UseBitMask=off  NumInputPorts=2  BitMask=bin2dec('11011001')  BitMaskRealWorld=Stored Integer
  Data Type Conversion{,1,3..4,6..7} (6 alike) : DataTypeConversion  OutDataTypeStr=uint16
  Data Type Conversion2 : DataTypeConversion  OutDataTypeStr=int16
  Data Type Conversion5 : DataTypeConversion  OutDataTypeStr=int16
  Data Type Conversion8 : DataTypeConversion  OutDataTypeStr=int16
  Shift Arithmetic : ArithShift  BitShiftNumber=-8
  Shift Arithmetic1 : ArithShift  BitShiftNumber=-8
  Shift Arithmetic2 : ArithShift  BitShiftNumber=-8
  value_ax : Outport
  value1_ay : Outport  Port=2
  value2_az : Outport  Port=3
  wires:
  MSB_ax/1 -> Data Type Conversion/1
  "LSB_ax "/1 -> Data Type Conversion1/1
  Data Type Conversion1/1 -> Shift Arithmetic/1
  Data Type Conversion/1 -> Bitwise Operator/2
  Bitwise Operator/1 -> Data Type Conversion2/1
  Shift Arithmetic/1 -> Bitwise Operator/1
  Data Type Conversion2/1 -> value_ax/1
  MSB_ay/1 -> Data Type Conversion3/1
  LSB_ay/1 -> Data Type Conversion4/1
  Data Type Conversion4/1 -> Shift Arithmetic1/1
  Data Type Conversion3/1 -> Bitwise Operator1/2
  Bitwise Operator1/1 -> Data Type Conversion5/1
  Shift Arithmetic1/1 -> Bitwise Operator1/1
  Data Type Conversion5/1 -> value1_ay/1
  MSB_az/1 -> Data Type Conversion6/1
  LSB_az/1 -> Data Type Conversion7/1
  Data Type Conversion7/1 -> Shift Arithmetic2/1
  Data Type Conversion6/1 -> Bitwise Operator2/2
  Bitwise Operator2/1 -> Data Type Conversion8/1
  Shift Arithmetic2/1 -> Bitwise Operator2/1
  Data Type Conversion8/1 -> value2_az/1

== system CubeX_LQR_2D/READ ACC AND GYRO WITH SPI/USE THIS ONE!!2 ==
  "Gyro_Zout_High " : Inport
  Gyro_Zout_Low : Inport  Port=2
  Bitwise Operator : simulink/Logic and Bit Operations/Bitwise Operator  logicop=OR  UseBitMask=off  NumInputPorts=2  BitMask=bin2dec('11011001')  BitMaskRealWorld=Stored Integer
  Data Type Conversion : DataTypeConversion  OutDataTypeStr=uint16
  Data Type Conversion1 : DataTypeConversion  OutDataTypeStr=uint16
  Shift Arithmetic : ArithShift  BitShiftNumber=-8
  Gyro_Zout : Outport
  wires:
  Gyro_Zout_Low/1 -> Data Type Conversion/1
  "Gyro_Zout_High "/1 -> Data Type Conversion1/1
  Data Type Conversion1/1 -> Shift Arithmetic/1
  Data Type Conversion/1 -> Bitwise Operator/2
  Shift Arithmetic/1 -> Bitwise Operator/1
  Bitwise Operator/1 -> Gyro_Zout/1

== system CubeX_LQR_2D/READ ACC AND GYRO WITH SPI/USE THIS ONE!!3 ==
  "Gyro_Zout_High " : Inport
  Gyro_Zout_Low : Inport  Port=2
  Bitwise Operator : simulink/Logic and Bit Operations/Bitwise Operator  logicop=OR  UseBitMask=off  NumInputPorts=2  BitMask=bin2dec('11011001')  BitMaskRealWorld=Stored Integer
  Data Type Conversion : DataTypeConversion  OutDataTypeStr=uint16
  Data Type Conversion1 : DataTypeConversion  OutDataTypeStr=uint16
  Shift Arithmetic : ArithShift  BitShiftNumber=-8
  Gyro_Zout : Outport
  wires:
  Gyro_Zout_Low/1 -> Data Type Conversion/1
  "Gyro_Zout_High "/1 -> Data Type Conversion1/1
  Data Type Conversion1/1 -> Shift Arithmetic/1
  Data Type Conversion/1 -> Bitwise Operator/2
  Shift Arithmetic/1 -> Bitwise Operator/1
  Bitwise Operator/1 -> Gyro_Zout/1

== system CubeX_LQR_2D/READ ACC AND GYRO WITH SPI/USE THIS ONE!!4 ==
  "Gyro_Zout_High " : Inport
  Gyro_Zout_Low : Inport  Port=2
  Bitwise Operator : simulink/Logic and Bit Operations/Bitwise Operator  logicop=OR  UseBitMask=off  NumInputPorts=2  BitMask=bin2dec('11011001')  BitMaskRealWorld=Stored Integer
  Data Type Conversion : DataTypeConversion  OutDataTypeStr=uint16
  Data Type Conversion1 : DataTypeConversion  OutDataTypeStr=uint16
  Shift Arithmetic : ArithShift  BitShiftNumber=-8
  Gyro_Zout : Outport
  wires:
  Gyro_Zout_Low/1 -> Data Type Conversion/1
  "Gyro_Zout_High "/1 -> Data Type Conversion1/1
  Data Type Conversion1/1 -> Shift Arithmetic/1
  Data Type Conversion/1 -> Bitwise Operator/2
  Shift Arithmetic/1 -> Bitwise Operator/1
  Bitwise Operator/1 -> Gyro_Zout/1

== system CubeX_LQR_2D/Read IMU/Accelometer Gyroscope I2C1 ==
  SlvAddr MPU9250 : Inport
  MPU9250 Init : Subsystem
  Read Accelometer and Gyroscope Data : Subsystem
  acc : Outport
  gyro : Outport  Port=2
  wires:
  SlvAddr MPU9250/1 -> Read Accelometer and Gyroscope Data/1(SlvAddr), MPU9250 Init/1(SlvAddr)
  Read Accelometer and Gyroscope Data/1(acc) -> acc/1
  Read Accelometer and Gyroscope Data/2(gyro) -> gyro/1
  MPU9250 Init/1(SETUP_READY) -> Read Accelometer and Gyroscope Data/Enable

== system CubeX_LQR_2D/Read IMU/Accelometer Gyroscope I2C3 ==
  SlvAddr MPU9250 : Inport
  MPU9250 Init : Subsystem
  Read Accelometer and Gyroscope Data : Subsystem
  acc : Outport
  gyro : Outport  Port=2
  wires:
  SlvAddr MPU9250/1 -> Read Accelometer and Gyroscope Data/1(SlvAddr), MPU9250 Init/1(SlvAddr)
  Read Accelometer and Gyroscope Data/1(acc) -> acc/1
  Read Accelometer and Gyroscope Data/2(gyro) -> gyro/1
  MPU9250 Init/1(SETUP_READY) -> Read Accelometer and Gyroscope Data/Enable
